simulink model "switch_case_action_subsystem"  (R2018b)
settings: Solver=FixedStepDiscrete  StartTime=0.0  StopTime=10.0  FixedStep=0.2  RelTol=1e-3
libraries: simulink x4
settings Model: Creator=marwan  LastModifiedBy=marwan

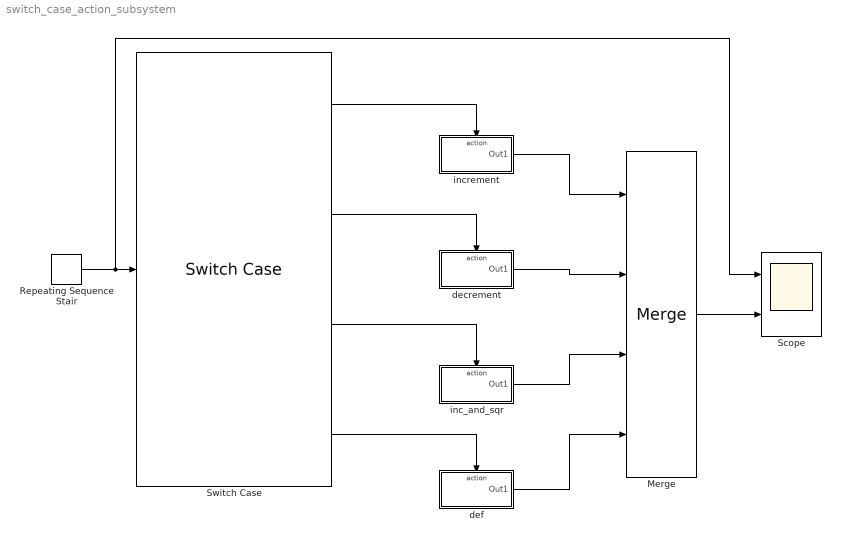
== system switch_case_action_subsystem ==
  Merge : Merge  Inputs=4
  Repeating Sequence Stair : simulink/Sources/Repeating Sequence Stair  OutValues=[1 1 1 1 1 3 3 3 3 3 2 2 2 2 2 4 4 4 4 4 6 6 6 6 6]  tsamp=-1  OutMin=[]  OutMax=[]  OutDataTypeStr=double  OutputDataTypeScalingMode=double  OutDataType=fixdt(0,8)  ConRadixGroup=Best Precision: Vector-wise  OutScaling=2^-12
  Scope : Scope  NumInputPorts=2
  Switch Case : SwitchCase  CaseConditions={1,2,[3,4]}
  decrement : Subsystem  TreatAsAtomicUnit=on
  def : Subsystem  TreatAsAtomicUnit=on
  inc_and_sqr : Subsystem  TreatAsAtomicUnit=on
  increment : Subsystem  TreatAsAtomicUnit=on
  wires:
  Switch Case/1 -> increment/Action
  Switch Case/2 -> decrement/Action
  Switch Case/3 -> inc_and_sqr/Action
  Switch Case/4 -> def/Action
  Repeating Sequence Stair/1 -> Scope/1, Switch Case/1
  increment/1(Out1) -> Merge/1
  decrement/1(Out1) -> Merge/2
  inc_and_sqr/1(Out1) -> Merge/3
  def/1(Out1) -> Merge/4
  Merge/1 -> Scope/2

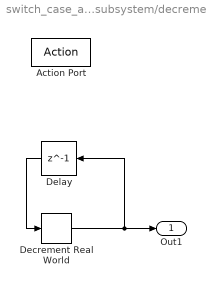
== system switch_case_action_subsystem/decrement ==
  Action Port : ActionPort  ActionType=case
  Decrement Real World : simulink/Additional Math & Discrete/Additional Math: Increment - Decrement/Decrement Real World
      settings: SourceProductName=Simulink  SourceProductBaseCode=SL
  Delay : Delay  DelayLength=1  InitialCondition=10
  Out1 : Outport
  wires:
  Decrement Real World/1 -> Delay/1, Out1/1
  Delay/1 -> Decrement Real World/1

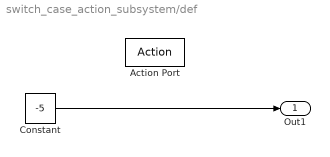
== system switch_case_action_subsystem/def ==
  Action Port : ActionPort  ActionType=default
  Constant : Constant  Value=-5
  Out1 : Outport
  wires:
  Constant/1 -> Out1/1

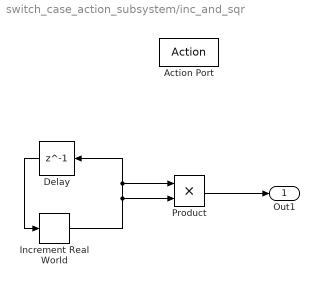
== system switch_case_action_subsystem/inc_and_sqr ==
  Action Port : ActionPort  ActionType=case
  Delay : Delay  DelayLength=1
  Increment Real World : simulink/Additional Math & Discrete/Additional Math: Increment - Decrement/Increment Real World
      settings: SourceProductName=Simulink  SourceProductBaseCode=SL
  Product : Product
  Out1 : Outport
  wires:
  Increment Real World/1 -> Product/2, Product/1, Delay/1
  Delay/1 -> Increment Real World/1
  Product/1 -> Out1/1

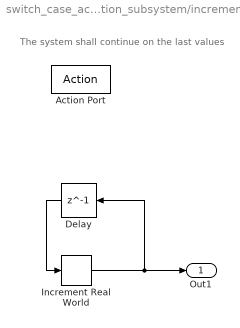
== system switch_case_action_subsystem/increment ==
  note: The system shall continue on the last values
  Action Port : ActionPort  ActionType=case
  Delay : Delay  DelayLength=1
  Increment Real World : simulink/Additional Math & Discrete/Additional Math: Increment - Decrement/Increment Real World
      settings: SourceProductName=Simulink  SourceProductBaseCode=SL
  Out1 : Outport
  wires:
  Increment Real World/1 -> Delay/1, Out1/1
  Delay/1 -> Increment Real World/1
